simulink model "lab03_1"  (R2025a)
settings: Solver=VariableStepAuto  StartTime=0.0  StopTime=500  RelTol=1e-4
settings Model: Creator=razrab-ytka  LastModifiedBy=grigorijtomczuk
settings SolverCC: AlgebraicLoopSolver=TrustRegion
settings DebuggingCC: ArithmeticOperatorsInVariantConditions=warning
settings SFSimCC: CustomCodeUndefinedFunction=UseInterfaceOnly
settings RTWCC: GPUComputeCapability=3.5
settings CodeAppCC: StateflowObjectComments=on

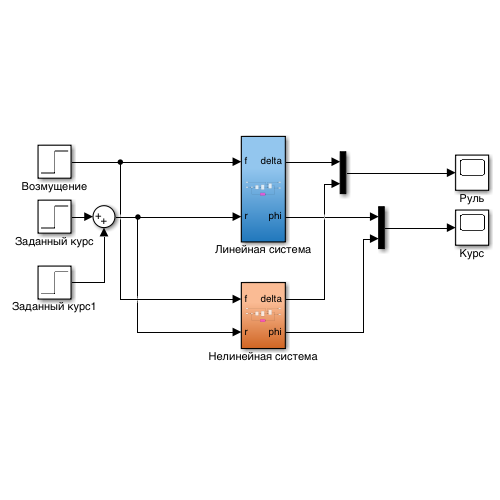
[thumbnail: Simulink's stored preview of the top-level diagram]
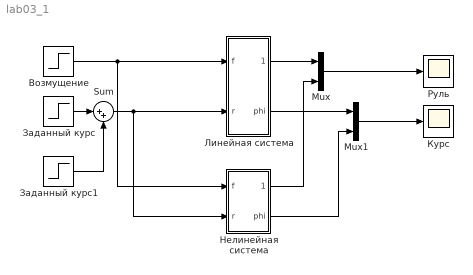
== system lab03_1 ==
  Mux : Mux  Inputs=2
  Mux1 : Mux  Inputs=2
  Sum : Sum  Inputs=|++
  Возмущение : Step  Time=0  After=0  SampleTime=0
  Заданный курс : Step  Time=10  After=37.5  SampleTime=0
  Заданный курс1 : Step  Time=40  After=37.5  SampleTime=0
  Курс : Scope
      settings: ActiveDisplayYMinimum=-14.173581654364332  ActiveDisplayYMaximum=127.56223488927903
  Линейная система : Subsystem
  Нелинейная система : Subsystem
  Руль : Scope
      settings: ActiveDisplayYMinimum=-27.52824982617058  ActiveDisplayYMaximum=45.407563064074822
  wires:
  Возмущение/1 -> Нелинейная система/1(f), Линейная система/1(f)
  Линейная система/1(delta) -> Mux/1
  Линейная система/2(phi) -> Mux1/1
  Mux/1 -> Руль/1
  Mux1/1 -> Курс/1
  Нелинейная система/1(delta) -> Mux/2
  Нелинейная система/2(phi) -> Mux1/2
  Заданный курс1/1 -> Sum/2
  Заданный курс/1 -> Sum/1
  Sum/1 -> Нелинейная система/2(r), Линейная система/2(r)

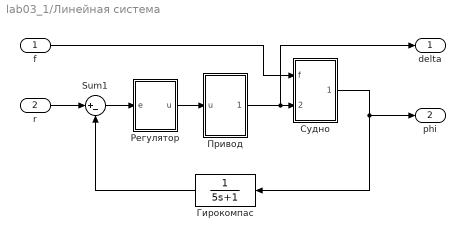
== system lab03_1/Линейная система ==
  f : Inport
  r : Inport  Port=2
  Sum1 : Sum  Inputs=|+-
  Гирокомпас : TransferFcn  Denominator=[5 1]
  Привод : Subsystem
  Регулятор : Subsystem
  Судно : Subsystem
  delta : Outport
  phi : Outport  Port=2
  wires:
  f/1 -> Судно/1(f)
  Sum1/1 -> Регулятор/1(e)
  r/1 -> Sum1/1
  Гирокомпас/1 -> Sum1/2
  Судно/1(phi) -> phi/1, Гирокомпас/1
  Регулятор/1(u) -> Привод/1(u)
  Привод/1(delta) -> delta/1, Судно/2(delta)

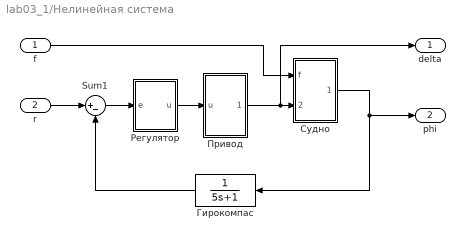
== system lab03_1/Нелинейная система ==
  f : Inport
  r : Inport  Port=2
  Sum1 : Sum  Inputs=|+-
  Гирокомпас : TransferFcn  Denominator=[5 1]
  Привод : Subsystem
  Регулятор : Subsystem
  Судно : Subsystem
  delta : Outport
  phi : Outport  Port=2
  wires:
  f/1 -> Судно/1(f)
  Sum1/1 -> Регулятор/1(e)
  r/1 -> Sum1/1
  Гирокомпас/1 -> Sum1/2
  Судно/1(phi) -> phi/1, Гирокомпас/1
  Регулятор/1(u) -> Привод/1(u)
  Привод/1(delta) -> delta/1, Судно/2(delta)

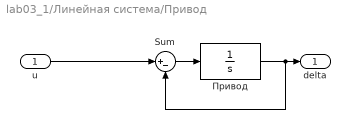
== system lab03_1/Линейная система/Привод ==
  u : Inport
  Sum : Sum  Inputs=|+-
  Привод : TransferFcn  Denominator=[1 0]
  delta : Outport
  wires:
  u/1 -> Sum/1
  Привод/1 -> Sum/2, delta/1
  Sum/1 -> Привод/1

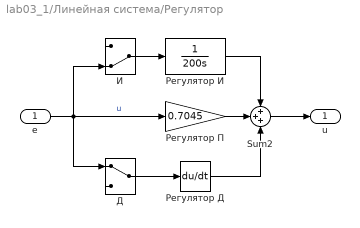
== system lab03_1/Линейная система/Регулятор ==
  e : Inport
  Sum2 : Sum  Inputs=+++
  Д : ManualSwitch
  И : ManualSwitch  CurrentSetting=0
  Регулятор Д : Derivative
  Регулятор И : TransferFcn  Denominator=[200 0]
  Регулятор П : Gain  Gain=0.7045
  u : Outport
  wires:
  Sum2/1 -> u/1
  И/1 -> Регулятор И/1
  Регулятор П/1 -> Sum2/2
  e/1 -> И/2, Д/1, Регулятор П/1  "u"
  Регулятор И/1 -> Sum2/1
  Д/1 -> Регулятор Д/1
  Регулятор Д/1 -> Sum2/3

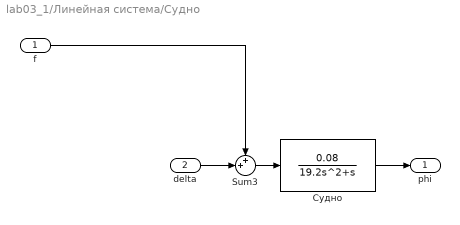
== system lab03_1/Линейная система/Судно ==
  f : Inport
  delta : Inport  Port=2
  Sum3 : Sum  Inputs=++|
  Судно : TransferFcn  Numerator=[0.08]  Denominator=[19.2 1 0]
  phi : Outport
  wires:
  Судно/1 -> phi/1
  delta/1 -> Sum3/2
  f/1 -> Sum3/1
  Sum3/1 -> Судно/1

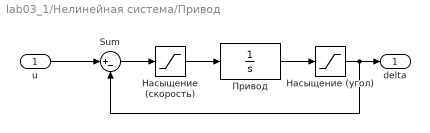
== system lab03_1/Нелинейная система/Привод ==
  u : Inport
  Sum : Sum  Inputs=|+-
  Насыщение (скорость) : Saturate  UpperLimit=3  LowerLimit=-3  ZeroCross=off
  Насыщение (угол) : Saturate  UpperLimit=30  LowerLimit=-30
  Привод : TransferFcn  Denominator=[1 0]
  delta : Outport
  wires:
  u/1 -> Sum/1
  Привод/1 -> Насыщение (угол)/1
  Насыщение (скорость)/1 -> Привод/1
  Sum/1 -> Насыщение (скорость)/1
  Насыщение (угол)/1 -> Sum/2, delta/1

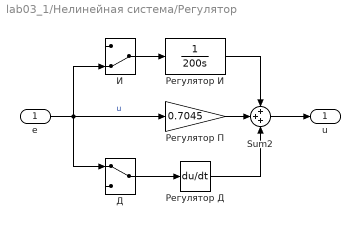
== system lab03_1/Нелинейная система/Регулятор ==
  e : Inport
  Sum2 : Sum  Inputs=+++
  Д : ManualSwitch
  И : ManualSwitch  CurrentSetting=0
  Регулятор Д : Derivative
  Регулятор И : TransferFcn  Denominator=[200 0]
  Регулятор П : Gain  Gain=0.7045
  u : Outport
  wires:
  Sum2/1 -> u/1
  И/1 -> Регулятор И/1
  Регулятор П/1 -> Sum2/2
  e/1 -> И/2, Д/1, Регулятор П/1  "u"
  Регулятор И/1 -> Sum2/1
  Д/1 -> Регулятор Д/1
  Регулятор Д/1 -> Sum2/3

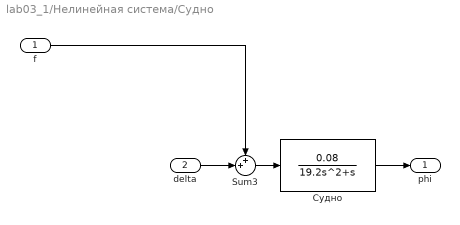
== system lab03_1/Нелинейная система/Судно ==
  f : Inport
  delta : Inport  Port=2
  Sum3 : Sum  Inputs=++|
  Судно : TransferFcn  Numerator=[0.08]  Denominator=[19.2 1 0]
  phi : Outport
  wires:
  Судно/1 -> phi/1
  delta/1 -> Sum3/2
  f/1 -> Sum3/1
  Sum3/1 -> Судно/1
